simulink model "Matlab_MPU9250"  (R2024b)
settings: Solver=FixedStepAuto  StartTime=0.0  StopTime=inf  FixedStep=Ts  RelTol=1e-3  EnableMultiTasking=on
InitFcn:
  | Ts=0.01;
  | Buff_len=500;
libraries: dspstat3 x2, arduinosensorlib x1
settings Model: ExtModeTrigDuration=2  Creator=Amin Danial  LastModifiedBy=Amin Danial
settings SolverCC: AutoInsertRateTranBlk=on
settings OptimizationCC: EnhancedBackFolding=on  PassReuseOutputArgsAs=Individual arguments  ZeroExternalMemoryAtStartup=off  ZeroInternalMemoryAtStartup=off  MaxStackSize=64  OptimizeBlockOrder=speed  DifferentSizesBufferReuse=on  OptimizationCustomize=off  EfficientTunableParamExpr=on
settings DebuggingCC: ParameterTunabilityLossMsg=error
settings HardwareCC: ProdBitPerInt=16  ProdBitPerPointer=16  ProdBitPerSizeT=16  ProdBitPerPtrDiffT=16  ProdLargestAtomicFloat=None  ProdWordSize=8  ProdHWDeviceType=Atmel->AVR
settings SFSimCC: MATLABDynamicMemAlloc=off
settings RTWCC: Description=Embedded Coder  SystemTargetFile=ert.tlc  HardwareBoard=Arduino Mega 2560  TemplateMakefile=ert_default_tmf  Toolchain=Arduino AVR  BuildConfiguration=Faster Runs  GPUComputeCapability=3.5
settings CodeAppCC: ForceParamTrailComments=on  IgnoreCustomStorageClasses=off  OperatorAnnotations=on  SimulinkDataObjDesc=on  SFDataObjDesc=on  InsertBlockDesc=on
settings ERTTargetCC: SupportContinuousTime=on  SupportVariableSizeSignals=on  ExtModeTransport=3  ExtModeStaticAlloc=on  ExtModeAutomaticAllocSize=off  ExtModeStaticAllocSize=2048  ExtModeMexFile=ext_xcp  ExtModeIntrfLevel=Level2 - Open  InlinedParameterPlacement=Hierarchical

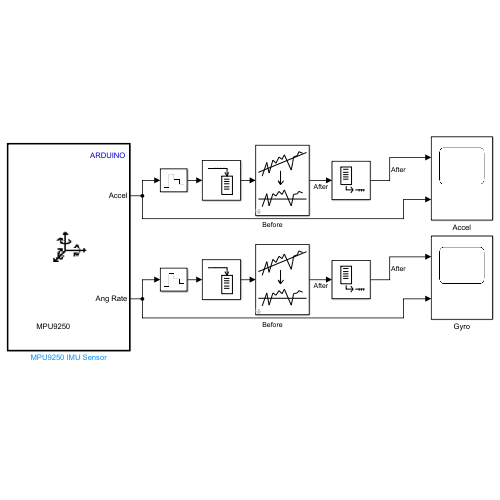
[thumbnail: Simulink's stored preview of the top-level diagram]
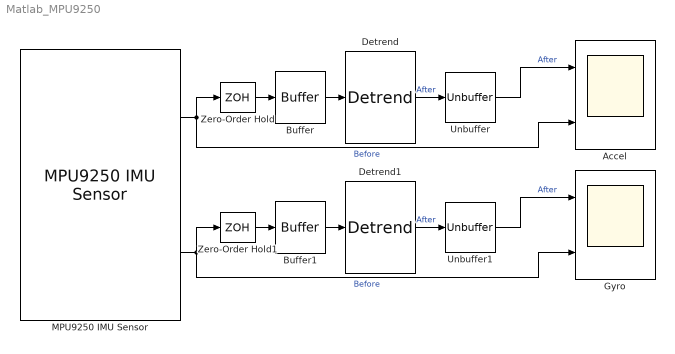
== system Matlab_MPU9250 ==
  Accel : Scope  NumInputPorts=2
  Buffer : Buffer  N=Buff_len  OutputFrames=off
  Buffer1 : Buffer  N=Buff_len  OutputFrames=off
  Detrend : dspstat3/Detrend
  Detrend1 : dspstat3/Detrend
  Gyro : Scope  NumInputPorts=2
  MPU9250 IMU Sensor : arduinosensorlib/MPU9250 IMU Sensor  I2CModule=0  SlaveAddress=0x68  Accel=on  AngularRate=on  Ak8963Field=off  Temperature=off  Status=off  EulerAngles=off  Quat=off  Timestamp=off  AccelRange=16G  Acceldlpf=10.2 Hz  GyroRange=2000 dps  Gyrodlpf=20 Hz  DmpOdr=200 Hz  spf=1  SampleTime=-1  QueueSizeFactor=1
      settings: SourceProductName=Sensors
  Unbuffer : Unbuffer
  Unbuffer1 : Unbuffer
  Zero-Order Hold : ZeroOrderHold  SampleTime=Ts
  Zero-Order Hold1 : ZeroOrderHold  SampleTime=Ts
  wires:
  MPU9250 IMU Sensor/1 -> Accel/2, Zero-Order Hold/1  "Before"
  Unbuffer/1 -> Accel/1  "After"
  Buffer/1 -> Detrend/1
  Zero-Order Hold/1 -> Buffer/1
  Detrend/1 -> Unbuffer/1  "After"
  Zero-Order Hold1/1 -> Buffer1/1
  Buffer1/1 -> Detrend1/1
  Detrend1/1 -> Unbuffer1/1  "After"
  MPU9250 IMU Sensor/2 -> Gyro/2, Zero-Order Hold1/1  "Before"
  Unbuffer1/1 -> Gyro/1  "After"
